simulink model "mReadMask"  (R2021a)
settings: Solver=FixedStepAuto  StartTime=0.0  StopTime=inf  RelTol=1e-3  EnableMultiTasking=on
settings Model: SILPILModeSetting=veronly  ExtModeTrigDuration=2  Creator=angelo  LastModifiedBy=angelo
settings OptimizationCC: EnhancedBackFolding=on  PassReuseOutputArgsAs=Individual arguments  ZeroExternalMemoryAtStartup=off  ZeroInternalMemoryAtStartup=off  MaxStackSize=64  OptimizeBlockOrder=speed  DifferentSizesBufferReuse=on  OptimizationCustomize=off  EfficientTunableParamExpr=on
settings DebuggingCC: ParameterTunabilityLossMsg=error
settings HardwareCC: ProdBitPerInt=16  ProdBitPerPointer=16  ProdBitPerSizeT=16  ProdBitPerPtrDiffT=16  ProdLargestAtomicFloat=None  ProdWordSize=8  ProdHWDeviceType=Atmel->AVR
settings SFSimCC: MATLABDynamicMemAlloc=off
settings RTWCC: SystemTargetFile=ert.tlc  HardwareBoard=Arduino Mega 2560  TemplateMakefile=ert_default_tmf  Toolchain=Arduino AVR  BuildConfiguration=Faster Runs
settings CodeAppCC: ForceParamTrailComments=on  IgnoreCustomStorageClasses=off  OperatorAnnotations=on  SimulinkDataObjDesc=on  SFDataObjDesc=on  InsertBlockDesc=on
settings ERTTargetCC: SupportContinuousTime=on  SupportVariableSizeSignals=on  ExtModeStaticAllocSize=2048

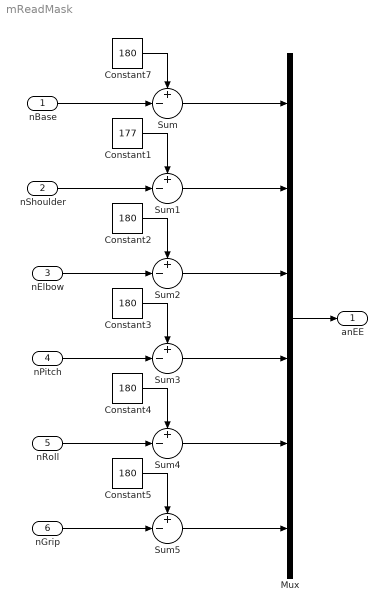
== system mReadMask ==
  nBase : Inport  OutDataTypeStr=int32
  nShoulder : Inport  Port=2  OutDataTypeStr=int32
  nElbow : Inport  Port=3  OutDataTypeStr=int32
  nPitch : Inport  Port=4  OutDataTypeStr=int32
  nRoll : Inport  Port=5  OutDataTypeStr=int32
  nGrip : Inport  Port=6  OutDataTypeStr=int32
  Constant1 : Constant  Value=177
  Constant{2..5,7} (5 alike) : Constant  Value=180
  Mux : Mux  Inputs=6
  Sum{,1..5} (6 alike) : Sum  Inputs=+-|
  anEE : Outport
  wires:
  Sum4/1 -> Mux/5
  nElbow/1 -> Sum2/2
  Constant3/1 -> Sum3/1
  Constant2/1 -> Sum2/1
  nBase/1 -> Sum/2
  Constant5/1 -> Sum5/1
  Sum1/1 -> Mux/2
  Constant1/1 -> Sum1/1
  nShoulder/1 -> Sum1/2
  Sum/1 -> Mux/1
  Constant7/1 -> Sum/1
  Constant4/1 -> Sum4/1
  Sum3/1 -> Mux/4
  Sum5/1 -> Mux/6
  Mux/1 -> anEE/1
  nPitch/1 -> Sum3/2
  Sum2/1 -> Mux/3
  nRoll/1 -> Sum4/2
  nGrip/1 -> Sum5/2
